simulink model "primer1_lec3"  (R2021b)
settings: Solver=ode45  StartTime=0.0  StopTime=0.5  RelTol=1e-3  EnableMultiTasking=on
settings Model: Creator=Alexander  LastModifiedBy=Admin
settings SolverCC: AlgebraicLoopSolver=TrustRegion
settings DataIOCC: LimitDataPoints=on  SaveFormat=Array  SignalLoggingSaveFormat=ModelDataLogs  ReturnWorkspaceOutputs=off
settings OptimizationCC: ExpressionDepthLimit=2147483647  InitFltsAndDblsToZero=on  LifeSpan=inf
settings DebuggingCC: SaveWithParameterizedLinksMsg=none  UnderspecifiedInitializationDetection=Classic  MergeDetectMultiDrivingBlocksExec=none  FcnCallInpInsideContextMsg=warning  StateNameClashWarn=warning  SFUnexpectedBacktrackingDiag=warning  SFNoUnconditionalDefaultTransitionDiag=warning  SFExecutionAtInitializationDiag=none  SFMachineParentedDataDiag=warning  ArithmeticOperatorsInVariantConditions=warning
settings HardwareCC: ProdBitPerPointer=32  ProdBitPerSizeT=32  ProdBitPerPtrDiffT=32  ProdLargestAtomicFloat=None  ProdIntDivRoundTo=Undefined  ProdEndianess=Unspecified  ProdWordSize=32  ProdHWDeviceType=32-bit Generic
settings ModelReferenceCC: PropagateSignalLabelsOutOfModel=off
settings CodeAppCC: StateflowObjectComments=on
settings GRTTargetCC: TargetFcnLib=ansi_tfl_tmw.mat  TargetLangStandard=C89/C90 (ANSI)  CombineOutputUpdateFcns=off  GRTInterface=on
settings ConfigComp: CovMetricSettings=dw  CovSaveCumulativeToWorkspaceVar=on  CovSaveSingleToWorkspaceVar=on

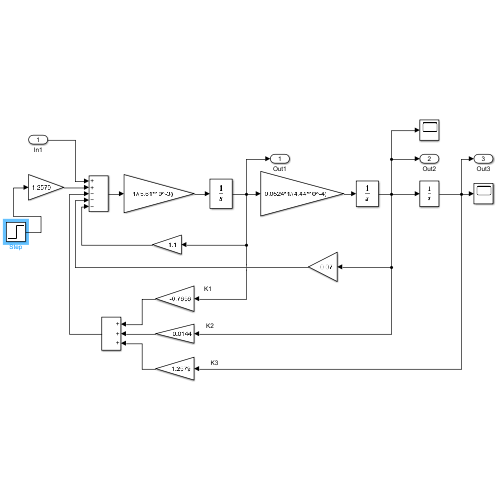
[thumbnail: Simulink's stored preview of the top-level diagram]
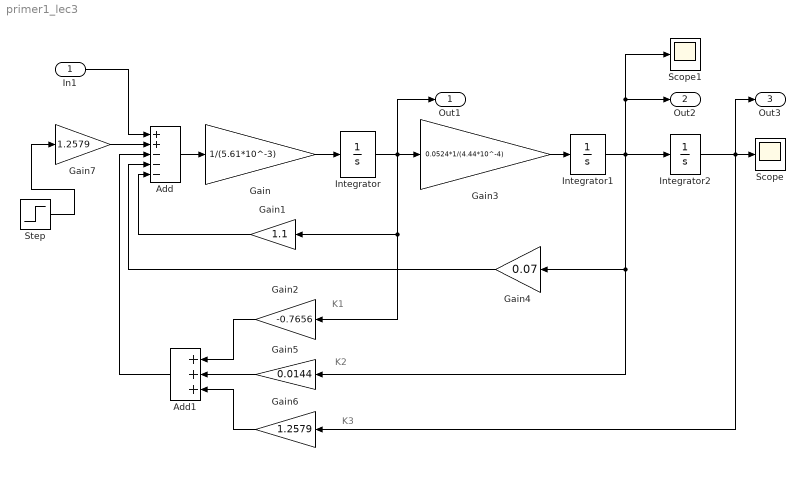
== system primer1_lec3 ==
  note: K3
  note: K2
  note: K1
  In1 : Inport
  Add : Sum  Inputs=++---
  Add1 : Sum  Inputs=+++
  Gain : Gain  Gain=1/(5.61*10^-3)
  Gain1 : Gain  Gain=1.1
  Gain2 : Gain  Gain=-0.7656
  Gain3 : Gain  Gain=0.0524*1/(4.44*10^-4)
  Gain4 : Gain  Gain=0.07
  Gain5 : Gain  Gain=0.0144
  Gain6 : Gain  Gain=1.2579
  Gain7 : Gain  Gain=1.2579
  Integrator : Integrator
  Integrator1 : Integrator
  Integrator2 : Integrator
  Scope : Scope
  Scope1 : Scope
  Step : Step  Time=0  SampleTime=0
  Out1 : Outport
  Out2 : Outport  Port=2
  Out3 : Outport  Port=3
  wires:
  Gain3/1 -> Integrator1/1
  Integrator1/1 -> Scope1/1, Out2/1, Integrator2/1, Gain5/1, Gain4/1
  Integrator/1 -> Out1/1, Gain1/1, Gain2/1, Gain3/1
  Gain/1 -> Integrator/1
  Add/1 -> Gain/1
  Gain1/1 -> Add/5
  Gain4/1 -> Add/4
  Integrator2/1 -> Out3/1, Gain6/1, Scope/1
  Step/1 -> Gain7/1
  In1/1 -> Add/1
  Gain2/1 -> Add1/1
  Gain6/1 -> Add1/3
  Gain5/1 -> Add1/2
  Add1/1 -> Add/3
  Gain7/1 -> Add/2
